simulink model "P3s"  (R2015b)
settings: Solver=VariableStepAuto  StartTime=0.0  StopTime=20  RelTol=1e-3
libraries: fl_lib x13, nesl_utility x6
settings Model: Creator=xmax1946  LastModifiedBy=xmax1946

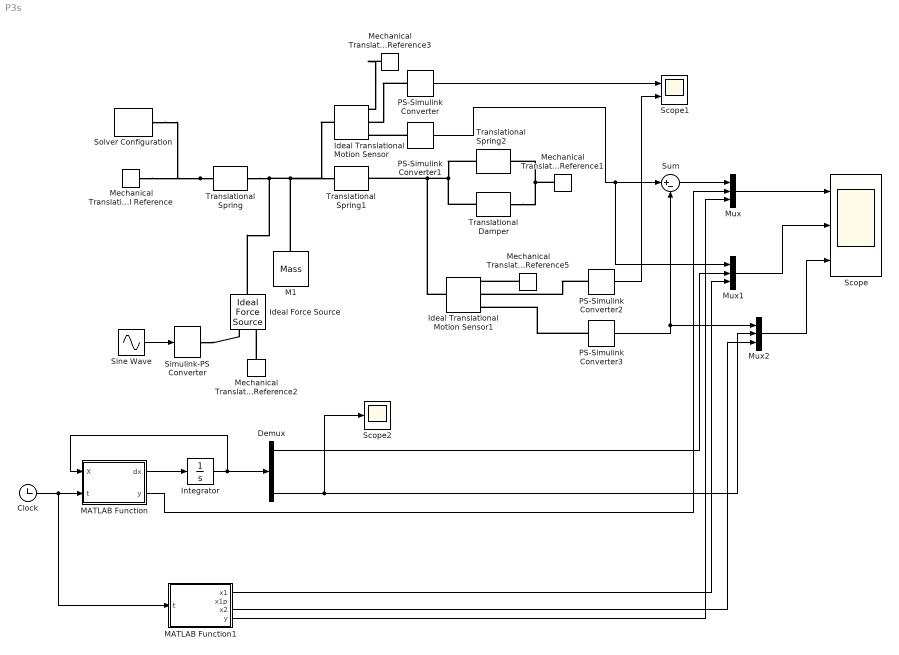
== system P3s ==
  Clock : Clock
  Demux : Demux  Outputs=3
  Ideal Force Source : fl_lib/Mechanical/Mechanical Sources/Ideal Force Source
  Ideal Translational Motion Sensor : fl_lib/Mechanical/Mechanical Sensors/Ideal Translational Motion Sensor  offset=0 m
  Ideal Translational Motion Sensor1 : fl_lib/Mechanical/Mechanical Sensors/Ideal Translational Motion Sensor  offset=0 m
  Integrator : Integrator  InitialCondition=[0;0;0]
  M1 : fl_lib/Mechanical/Translational Elements/Mass  mass=10 kg  v_specify=on  v_priority=High  v=0 m/s  f_specify=off  f_priority=None  f=0 N
  MATLAB Function : MATLAB Function  TreatAsAtomicUnit=on
  MATLAB Function1 : MATLAB Function  TreatAsAtomicUnit=on
  Mechanical Translational Reference{,1..3,5} (5 alike) : fl_lib/Mechanical/Translational Elements/Mechanical Translational Reference
  Mux : Mux  Inputs=3
  Mux1 : Mux  Inputs=3
  Mux2 : Mux  Inputs=3
  PS-Simulink Converter{,1..3} (4 alike) : nesl_utility/PS-Simulink Converter  PhysicalDomain=network_engine_domain  SubClassName=ps_output  LeftPortType=input  RightPortType=output  PseudoPeriodic=off  Frequencies=[]  Unit=1  AffineConversion=off
  Scope : Scope  NumInputPorts=3
  Scope1 : Scope  NumInputPorts=2
  Scope2 : Scope
  Simulink-PS Converter : nesl_utility/Simulink-PS Converter  PhysicalDomain=network_engine_domain  SubClassName=ps_input  LeftPortType=input  RightPortType=output  PseudoPeriodic=off  Frequencies=[]  NoiseDistribution=none  NoiseParameters=[]  Unit=1  AffineConversion=off  InputFiltering=off  SimscapeFilterOrder=1  InputFilterTimeConstant=0.001  UdotUserProvided=1
  Sine Wave : Sin  SampleTime=0
  Solver Configuration : nesl_utility/Solver Configuration  PhysicalDomain=network_engine_domain  SubClassName=solver  LeftPortType=input  RightPortType=generic  Accelerate=off  Tones=[]  Harmonics=[]  SimulateNoise=off  Profile=off  UseLocalSampling=off  EnableSwitchedLinearOptims=on  FrequencyDomain=off  UseCCode=off  RelTol=0.001  AbsTol=1e-06  MinStep=1e-09  ToWorkspace=off  RevertToSquareIcSolve=off  NumHomotopyIterations=100  PhasorMode=off  PhasorModeNumHarmonics=1  DoDC=off  ResidualTolerance=1e-09  UseLocalSolver=off  LocalSolverChoice=NE_BACKWARD_EULER_ADVANCER  LocalSolverSampleTime=0.001  DoFixedCost=off  MaxNonlinIter=3  MaxModeIter=2  LinearAlgebra=Sparse  DelaysMemoryBudget=1024  AutomaticFiltering=on  FilteringTimeConstant=0.001
  Sum : Sum  Inputs=|+-
  Translational Damper : fl_lib/Mechanical/Translational Elements/Translational Damper  D=.5 N/(m/s)  v_specify=off  v_priority=None  v=0 m/s  f_specify=off  f_priority=None  f=0 N
  Translational Spring : fl_lib/Mechanical/Translational Elements/Translational Spring  spr_rate=2 N/m  v_specify=off  v_priority=None  v=0 m/s  f_specify=off  f_priority=None  f=0 N  x_specify=on  x_priority=High  x=0 m
  Translational Spring1 : fl_lib/Mechanical/Translational Elements/Translational Spring  spr_rate=1 N/m  v_specify=off  v_priority=None  v=0 m/s  f_specify=off  f_priority=None  f=0 N  x_specify=on  x_priority=High  x=0 m
  Translational Spring2 : fl_lib/Mechanical/Translational Elements/Translational Spring  spr_rate=.5 N/m  v_specify=off  v_priority=None  v=0 m/s  f_specify=off  f_priority=None  f=0 N  x_specify=on  x_priority=High  x=0 m
  wires:
  Sine Wave/1 -> Simulink-PS Converter/1
  PS-Simulink Converter1/1 -> Mux1/1, Sum/1
  PS-Simulink Converter3/1 -> Mux2/1, Sum/2
  Clock/1 -> MATLAB Function1/1(t), MATLAB Function/2(t)
  Integrator/1 -> Demux/1, MATLAB Function/1(X)
  MATLAB Function/1(dx) -> Integrator/1
  Sum/1 -> Mux/1
  Mux/1 -> Scope/1
  Demux/3 -> Scope2/1, Mux2/2
  Mux1/1 -> Scope/2
  Mux2/1 -> Scope/3
  PS-Simulink Converter2/1 -> Scope1/2
  MATLAB Function/2(y) -> Mux/2
  MATLAB Function1/1(x1) -> Mux1/3
  MATLAB Function1/3(x2) -> Mux2/3
  Demux/1 -> Mux1/2
  PS-Simulink Converter/1 -> Scope1/1
  MATLAB Function1/4(y) -> Mux/3
  connections:
  Translational Spring/LConn1 -- Mechanical Translational Reference/LConn1 -- Solver Configuration/RConn1
  Ideal Force Source/LConn1 -- Translational Spring/RConn1 -- Ideal Translational Motion Sensor/LConn1 -- Translational Spring1/LConn1 -- M1/LConn1
  Translational Spring2/LConn1 -- Translational Damper/LConn1 -- Ideal Translational Motion Sensor1/LConn1 -- Translational Spring1/RConn1
  Mechanical Translational Reference3/LConn1 -- Ideal Translational Motion Sensor/RConn1
  Mechanical Translational Reference2/LConn1 -- Ideal Force Source/RConn2
  Mechanical Translational Reference1/LConn1 -- Translational Damper/RConn1 -- Translational Spring2/RConn1
  PS-Simulink Converter1/LConn1 -- Ideal Translational Motion Sensor/RConn3
  Mechanical Translational Reference5/LConn1 -- Ideal Translational Motion Sensor1/RConn1
  PS-Simulink Converter/LConn1 -- Ideal Translational Motion Sensor/RConn2
  PS-Simulink Converter3/LConn1 -- Ideal Translational Motion Sensor1/RConn3
  PS-Simulink Converter2/LConn1 -- Ideal Translational Motion Sensor1/RConn2
  Simulink-PS Converter/RConn1 -- Ideal Force Source/RConn1

== matlab function P3s/MATLAB Function1 ==
  data: x1 output; x1p output; x2 output; y output; t input
function [x1,x1p,x2,y] = fcn(t)
x1=0.000024447000534299612289796785289094*exp(-2.9781888183120855013344827821287*t) - 0.0034602076124567474048442906574394*cos(t) - 0.1314878892733564013840830449827*sin(t) + 0.27151062921957282867439002308629*exp(-0.010905590843957249332758608935638*t)*sin(0.48468881838889569804507542020527*t) + 0.0034357606119224477925544938721504*exp(-0.010905590843957249332758608935638*t)*cos(0.48468881838889569804507542020527*t);
x1p=0.0034602076124567474048442906574394*sin(t) - 0.00007280778363252068520107942437931*exp(-2.9781888183120855013344827821287*t) - 0.1314878892733564013840830449827*cos(t) - 0.0046262585833138454951496444703428*exp(-0.010905590843957249332758608935638*t)*sin(0.48468881838889569804507542020527*t) + 0.13156069705698892206928412440708*exp(-0.010905590843957249332758608935638*t)*cos(0.48468881838889569804507542020527*t);
x2=0.024221453287197231833910034602076*cos(t) + 0.0022416942726074866316249962676694*exp(-2.9781888183120855013344827821287*t) - 0.079584775086505190311418685121107*sin(t) + 0.17737642046148386317156230961807*exp(-0.010905590843957249332758608935638*t)*sin(0.48468881838889569804507542020527*t) - 0.026463147559804718465535030869746*exp(-0.010905590843957249332758608935638*t)*cos(0.48468881838889569804507542020527*t);
y=0.094134208758088965502827713468213*exp(-0.010905590843957249332758608935638*t)*sin(0.48468881838889569804507542020527*t) - 0.0022172472720731870193351994823803*exp(-2.9781888183120855013344827821287*t) - 0.051903114186851211072664359861592*sin(t) - 0.027681660899653979238754325259516*cos(t) + 0.029898908171727166258089524741896*exp(-0.010905590843957249332758608935638*t)*cos(0.48468881838889569804507542020527*t);

== matlab function P3s/MATLAB Function ==
  data: dx output; X input; y output; t input
function [dx,y] = fcn(X,t)
k1=2;
k2=1;
k3=.5;  
b1=.5;
m1=10;
A=[0,1,0;(-1/m1)*(k2+k1),0,k2/m1;k2/b1,0,-(k3+k2)/b1];
B=[0;1/m1;0];
C=[1,0,-1];
u=sin(t);
dx=A*X+B*u;
y=C*X;
